simulink model "Model_RB_APF_WF"  (R2024b)
settings: Solver=FixedStepAuto  StartTime=0.0  StopTime=90  FixedStep=UAVSampleTime  RelTol=1e-3
undefined symbols (not defined in the file): DroneMass, Gravity, Horizontal_Limits, Horizontal_Res, kD_pos, kD_vel, kI_pos, kI_vel, kP_pos, kP_vel, Lidar, MaxRange, N_filter, TopSpeed, UAV, Vertical_Limits, Vertical_Res, Waypoints
libraries: slpidlib x6, uavsimlib x4, robotcorelib x1, uavalgslib x1
(part 2 of 2)

== matlab function Model_RB_APF_WF/APF/RepulseWithVirtuals_V5 ==
  data: cloud input; virtuals input; virtualCount input; q input; del_U_rep output
function del_U_rep = repulsive(cloud, virtuals, virtualCount, q)

% Sort of 2 basic approaches. Define repulse in terms of either: ALL or CLOSEST obstacles

% Parameters
Q_star = 5;     % how far away we ignore obstacles at
eta = 0.03;    % how strongly we reppel from obstacles (how soon del_U_rep goes to infinity)
veta = 200;     % how strongly we reppel from virtual obstacles


del_U_rep = zeros(size(q));    % 3x1 vector

% Cloud Repulse
r_all = -cloud.';                          % 3xN
D_all = sqrt(sum(r_all.^2, 1));            % 1xN
in_range  = D_all <= Q_star & D_all > 0;       % 1xN logical
r_m   = r_all(:, in_range);                    % 3xM
D_m   = D_all(in_range);                       % 1xM
del_U_rep = del_U_rep + eta * sum((1./D_m - 1/Q_star) .* (1./D_m.^2) .* (r_m ./ D_m), 2);

% Virtuals Repulse
if virtualCount > 0
    v_r_all    = -(virtuals(1:virtualCount,:).' - q);
    v_D_all    = sqrt(sum(v_r_all.^2, 1));
    v_in_range = v_D_all <= Q_star & v_D_all > 0;
    v_r_m      = v_r_all(:, v_in_range);
    v_D_m      = v_D_all(v_in_range);
    del_U_rep  = del_U_rep + veta * sum((1./v_D_m - 1/Q_star) .* (1./v_D_m.^2) .* (v_r_m ./ v_D_m), 2);
end

== matlab function Model_RB_APF_WF/Vertical Constraint/MATLAB Function ==
  data: desired_pos input; constrained_pos output; current_waypoint input
function constrained_pos = constrainZ(desired_pos, current_waypoint)

constrained_pos = [desired_pos(1); desired_pos(2); current_waypoint(3)];

== matlab function Model_RB_APF_WF/Path Planning Data/MATLAB Function ==
  data: pts input; points output
function points = lidarToPoints(pts)

xLidar = reshape(pts(:,:,1),[],1);
yLidar = reshape(pts(:,:,2),[],1);
zLidar = reshape(pts(:,:,3),[],1);
    
points = [xLidar,yLidar,zLidar];    % Lidar points are in X,Y,Z order

== matlab function Model_RB_APF_WF/LML Indicators/LML_indicators ==
  settings: updateMethod=DISCRETE
  data: APF_pos input; APF_mag output; position input; target input; disp_1s output; t input; disp_3s output; dist2goal output
function [APF_mag, disp_1s, disp_3s, dist2goal] = LML_indicators(APF_pos, position, target, t)

Tmax = 180;

persistent pos_hist
persistent lastSec

if isempty(pos_hist)
    pos_hist = zeros(Tmax+1, 3);
    lastSec  = int32(-1);
end

% APF_mag 
APF_mag = norm(APF_pos(:) - position(:));

% Time and Pos_hist
sec = int32(floor(t));
if sec ~= lastSec && sec >= 0 && sec <= Tmax
    pos_hist(sec+1, :) = position(:).';
    lastSec = sec;
end

% Disp1s
if sec >= 1
    disp_1s = norm(position(:) - pos_hist(sec, :).');
else
    disp_1s = 0;
end

% Disp3s
if sec >= 3
    disp_3s = norm(position(:) - pos_hist(sec-2, :).');
else
    disp_3s = 0;
end

% Dist2goal
dist2goal = norm(target-position);

== matlab function Model_RB_APF_WF/Rule-Based Mode Switcher/RB mode manager ==
  settings: updateMethod=DISCRETE
  data: position input; flight_mode output; goal input; cloud input; APF_pos input; WF_pos input; t input; desired_pos output; Minima_list output; Minima_count output; critPoint_list output; critPoint_count output; APF_mag input; dist2goal input; d_1s input; d_3s input; theta_APF_WF input; d_closest_LM input; C_obs input
function [flight_mode, desired_pos, Minima_list, Minima_count, critPoint_list, critPoint_count] = modeManager(position, goal, cloud, APF_pos, WF_pos, t, APF_mag, dist2goal, d_1s, d_3s, theta_APF_WF, d_closest_LM, C_obs)

% Parameters

thresh_F_APF        = 3;  
thresh_d_goal       = 8;   
thresh_d_1s         = 0.5;
thresh_d_3s         = 1;

thresh_APF_WF_angle = 25;
thresh_LM_dist      = 2;
thresh_C_obs        = 0.5;

LMmax            = 100;     % max VOs
CPmax                = 100;     % max CPs

% Persistent variables
persistent mode
persistent LM_list
persistent LM_count
persistent CP_list
persistent CP_count

if isempty(mode)
    mode             = 1;
    LM_list          = zeros(LMmax, 3);
    LM_count         = 0;
    CP_list          = zeros(CPmax, 3);
    CP_count         = 0;
end


% Default outputs
flight_mode    = mode;
desired_pos    = APF_pos;
Minima_list    = LM_list;
Minima_count   = LM_count;
critPoint_list  = CP_list;
critPoint_count = CP_count;

% Dont start switching until we have a few seconds of data
if t<= 3
    return;
end

switch mode

    case 1  % APF mode

        desired_pos = APF_pos;
        
        % Crisp Rule Equivalent Switching Conditions

        LM_vote_force_goal = (APF_mag < thresh_F_APF) && ~(dist2goal < thresh_d_goal);  % rules 1-4
        LM_vote_move_1s    = d_1s < thresh_d_1s;                                        % rules 5-6
        LM_vote_move_3s    = d_3s < thresh_d_3s;                                        % rules 7-8

        LM_votes = LM_vote_force_goal + LM_vote_move_1s + LM_vote_move_3s;

        if LM_votes >= 3   % LM trigger condition
            disp("Local Minima Detected at t ="); disp(t);
            
            % Place LM at current Position
            LM_count = LM_count + 1;
            LM_list(LM_count, :) = position(:).';
            assignin('base', 'finalMinimaList',  LM_list);
            assignin('base', 'finalMinimaCount', LM_count);

            % Determine WF direction (left or right)
            forwardXY    = goal(1:2) - position(1:2);
            left_points  = 0;
            right_points = 0;
            n_points = size(cloud, 1);
            for i = 1:n_points
                point_dir_XY = cloud(i, 1:2);
                cross_z = forwardXY(1)*point_dir_XY(2) - point_dir_XY(1)*forwardXY(2);
                if cross_z > 0
                    left_points = left_points + 1;
                elseif cross_z < 0
                    right_points = right_points + 1;
                end
            end
            if left_points < right_points
                mode = 2;
            else
                mode = 3;
            end
        end

        flight_mode = mode;
        Minima_list = LM_list;
        Minima_count = LM_count;

    case {2, 3}  % WF mode

        desired_pos = WF_pos;
        
        % Crisp Rule Equivalent Switching Conditions
        CP_vote_angle   = theta_APF_WF < thresh_APF_WF_angle;   % rules 1-2
        CP_vote_LM_dist = ~(d_closest_LM < thresh_LM_dist);     % rule 3 (two-sided: far from LM votes CP)
        CP_vote_density = C_obs < thresh_C_obs;                 % rules 4-5

        CP_votes = CP_vote_angle + CP_vote_LM_dist + CP_vote_density;

        if CP_votes >= 3   % CP trigger condition
        disp("CP Detected at t ="); disp(t);
        %fprintf('CP t=%.3f | theta=%.1f d_LM=%.2f C_obs=%.2f | votes %d %d %d\n', ...
        %t, theta_APF_WF, d_closest_LM, C_obs, ...
        %int32(CP_vote_angle), int32(CP_vote_LM_dist), int32(CP_vote_density));

            CP_count = CP_count + 1;
            CP_list(CP_count, :) = position(:).';
            assignin('base', 'finalCPList',  CP_list);
            assignin('base', 'finalCPCount', CP_count);
            mode = 1;
        end

        flight_mode = mode;
        critPoint_list = CP_list;
        critPoint_count = CP_count;

    otherwise
        desired_pos = APF_pos;
        flight_mode = mode;
end

== matlab function Model_RB_APF_WF/Controller/Attitude Control/Multirotor Acceleration Control ==
  data: acc input; roll output; pitch output; thrust output; yaw input; DroneMass parameter; Gravity parameter
function [roll, pitch, thrust] = accControl(acc, yaw, DroneMass, Gravity)

    xddot = acc(1);
    yddot = acc(2);
    zddot = acc(3);
    
    pitch = atan2((-xddot*cos(yaw)-yddot*sin(yaw)), ( -zddot + Gravity));
    roll = atan2(((-xddot*sin(yaw)+yddot*cos(yaw))*cos(pitch)), (-zddot+Gravity));
    
    roll_limit = 25*pi/180;
    pitch_limit = 25*pi/180;
    
    roll = min(roll_limit, max(-roll_limit, roll));
   
    pitch = min(pitch_limit, max(-pitch_limit, pitch));
    
    thrust = DroneMass*(-zddot+Gravity)/(cos(pitch)*cos(roll));
end

== matlab function Model_RB_APF_WF/Path Planning Data/VOActivator_V5 ==
  settings: updateMethod=DISCRETE
  data: Minima_list input; Minima_count input; position input; Virtuals_list output; flight_mode input; Virtuals_count output; t input
function [Virtuals_list, Virtuals_count] = VOActivator(Minima_list, Minima_count, position, flight_mode, t)

activation_dist = 3;
maxVO = 100;

persistent VO_list
persistent VO_count
persistent next_to_check
persistent was_in_WF

if isempty(VO_list)
    VO_list      = zeros(maxVO, 3);
    VO_count     = 0;
    next_to_check = 1;
    was_in_WF     = false(maxVO, 1);

    % Pass to workspace at least once
    assignin('base', 'finalVOList',  VO_list);
    assignin('base', 'finalVOCount', VO_count);
    
end

% Mark all current unactivated minima as having been in WF
if flight_mode == 2 || flight_mode == 3
    was_in_WF(next_to_check:Minima_count) = true;
end

% Check unactivated minima for activation
for i = next_to_check:Minima_count
    d = norm(position(:) - Minima_list(i,:).');
    if d > activation_dist || (flight_mode == 1 && was_in_WF(i))
        % VO is activated
        % disp("VO Activated at t ="); disp(t);
        VO_count = VO_count + 1;
        VO_list(VO_count, :) = Minima_list(i,:);
        next_to_check = i + 1;
        % Update VO list in workspace
        assignin('base', 'finalVOList',  VO_list);
        assignin('base', 'finalVOCount', VO_count);
    end
end

Virtuals_list  = VO_list;
Virtuals_count = VO_count;
